simulink model "PIDSimulink"  (R2019a)
settings: Solver=FixedStepAuto  StartTime=0.0  StopTime=100  FixedStep=1e-4  RelTol=1e-3
libraries: simulink x2
settings Model: Creator=luisg  LastModifiedBy=luisg

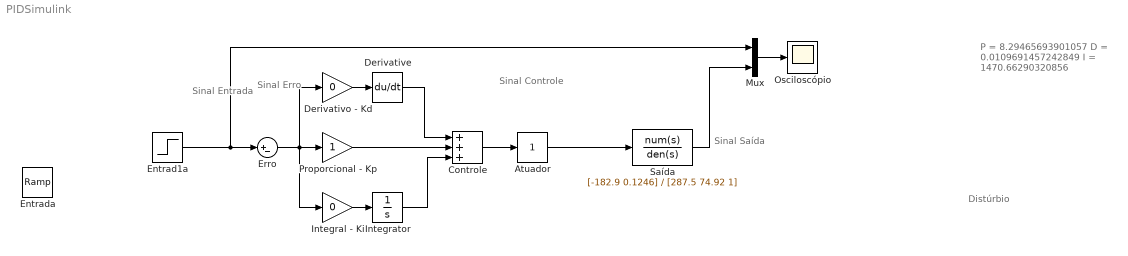
== system PIDSimulink ==
  note: P = 8.29465693901057
      | D = 0.0109691457242849
      | I = 1470.66290320856
  note: Sinal
      | Entrada
  note: Sinal
      | Erro
  note: Distúrbio
  note: Sinal
      | Controle
  note: Sinal
      | Saída
  Atuador : simulink/Math Operations/Slider Gain  gain=1  low=0  high=2
  Controle : Sum  Inputs=+++
  Derivative : Derivative
  Derivativo - Kd : Gain  Gain=0
  Entrad1a : Step  Time=0  SampleTime=0
  Entrada : simulink/Sources/Ramp  slope=1  start=0  InitialOutput=0
  Erro : Sum  Inputs=|+-
  Integral - Ki : Gain  Gain=0
  Integrator : Integrator
  Mux : Mux  Inputs=2
  Osciloscópio : Scope
  Proporcional - Kp : Gain
  Saída : TransferFcn  Numerator=[-182.9 0.1246]  Denominator=[287.5 74.92 1]  ContinuousStateAttributes='Planta'
  wires:
  Mux/1 -> Osciloscópio/1
  Erro/1 -> Integral - Ki/1, Derivativo - Kd/1, Proporcional - Kp/1
  Saída/1 -> Mux/2
  Entrad1a/1 -> Mux/1, Erro/1
  Integral - Ki/1 -> Integrator/1
  Controle/1 -> Atuador/1
  Derivativo - Kd/1 -> Derivative/1
  Proporcional - Kp/1 -> Controle/2
  Integrator/1 -> Controle/3
  Derivative/1 -> Controle/1
  Atuador/1 -> Saída/1
